simulink model "model"  (R2023b)
settings: Solver=FixedStepAuto  StartTime=0.0  StopTime=20  FixedStep=0.001  RelTol=1e-3
values from neighbouring files (symbols this model uses):
  A = [0 1; -15 6]    [calc.m]
  A_M = [0 1; -omega_0^2 -2*omega_0]    [calc.m]
  b = [0; 2]    [calc.m]
  b_M = [0; omega_0^2]    [calc.m]
  gamma = 10    [calc.m]
  P = [5 2; 2 1]    [calc.m]
  theta = ((A_M(2, :) - A(2, :)) / b(2)).'    [calc.m]
settings Model: Creator=Катя  LastModifiedBy=Катя

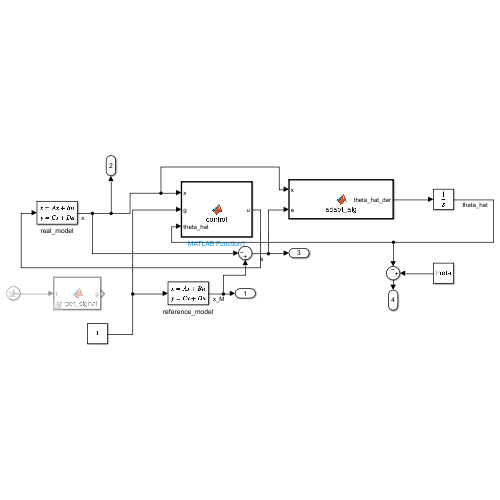
[thumbnail: Simulink's stored preview of the top-level diagram]
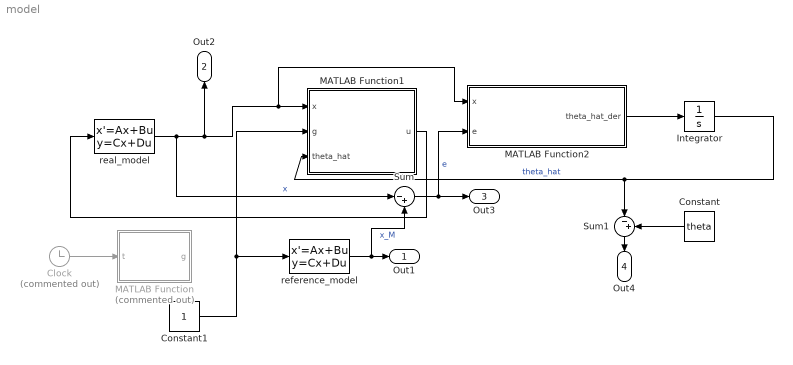
== system model ==
  Clock : Clock  Commented=on
  Constant : Constant  Value=theta
  Constant1 : Constant
  Integrator : Integrator
  MATLAB Function : MATLAB Function  Commented=on  TreatAsAtomicUnit=on
  MATLAB Function1 : MATLAB Function  TreatAsAtomicUnit=on
  MATLAB Function2 : MATLAB Function  TreatAsAtomicUnit=on
  Sum : Sum  Inputs=|-+
  Sum1 : Sum  Inputs=|-+
  real_model : StateSpace  A=A  B=b  C=[1 0; 0 1]  D=[0; 0]  InitialCondition=[0; 0]
  reference_model : StateSpace  A=A_M  B=b_M  C=[1 0; 0 1]  D=[0; 0]  InitialCondition=0
  Out1 : Outport
  Out2 : Outport  Port=2
  Out3 : Outport  Port=3
  Out4 : Outport  Port=4
  wires:
  reference_model/1 -> Sum/2, Out1/1  "x_M"
  Clock/1 -> MATLAB Function/1(t)
  Constant1/1 -> MATLAB Function1/2(g), reference_model/1
  real_model/1 -> Sum/1, Out2/1, MATLAB Function2/1(x), MATLAB Function1/1(x)  "x"
  MATLAB Function1/1(u) -> real_model/1
  Sum/1 -> MATLAB Function2/2(e), Out3/1  "e"
  MATLAB Function2/1(theta_hat_der) -> Integrator/1
  Integrator/1 -> Sum1/1, MATLAB Function1/3(theta_hat)  "theta_hat"
  Sum1/1 -> Out4/1
  Constant/1 -> Sum1/2

== matlab function model/MATLAB Function1 ==
  data: x input; u output; g input; kappa parameter; theta_hat input
function u = control(x, g, kappa, theta_hat)
    u = theta_hat.' * x + g / kappa;
end

== matlab function model/MATLAB Function ==
  data: t input; g output
function g = target_signal(t)
    g = 7 * sign(cos(0.9 * t)) + 8;
end

== matlab function model/MATLAB Function2 ==
  data: x input; theta_hat_der output; e input; gamma parameter; b parameter; P parameter
function theta_hat_der = adapt_alg(x, e, gamma, b, P)
    theta_hat_der = gamma * x * b.' * P * e;
end
